simulink model "Versuch_1 (1)"  (R2022b)
settings: Solver=VariableStepAuto  StartTime=0.0  StopTime=inf  MaxStep=0.00001  RelTol=1e-3
libraries: simulink_extras x2, simulink x2
settings Model: Creator=mouaz  LastModifiedBy=mouaz

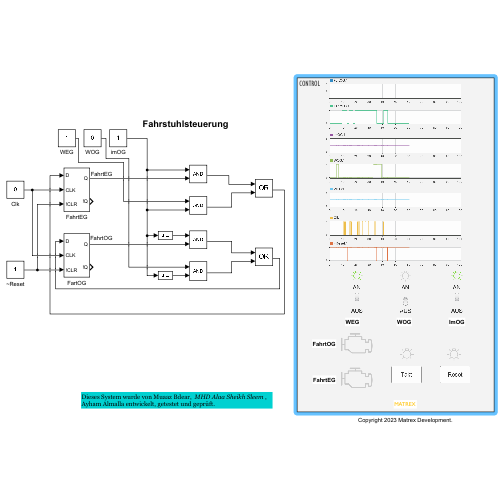
[thumbnail: Simulink's stored preview of the top-level diagram]
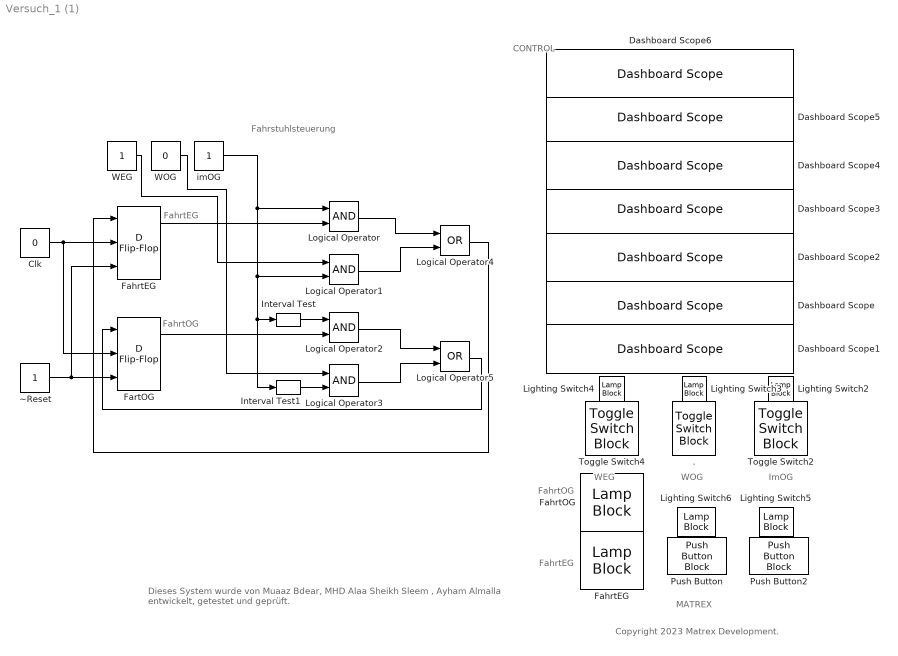
== system Versuch_1 (1) ==
  note: MATREX
  note: FahrtOG
  note: WEG
  note: FahrtEG
  note: FahrtOG
  note: WOG
  note: ImOG
  note: FahrtEG
  note: CONTROL
  note: Fahrstuhlsteuerung
  note: Copyright 2023 Matrex Development.
  note: Dieses System wurde von Muaaz Bdear, MHD Alaa Sheikh Sleem , Ayham Almalla entwickelt, getestet und geprüft.
  " FahrtEG" : LampBlock  LabelPosition=Hide  Icon=Engine
  . : ToggleSwitchBlock  LabelPosition=Hide
      settings: Values={{'AUS', 'AN'}, [0 1]}
  Clk : Constant  Value=0
  Dashboard Scope{,1..6} (7 alike) : DashboardScope
  FahrtEG : simulink_extras/Flip Flops/D Flip-Flop
  FahrtOG : LampBlock  LabelPosition=Hide  Icon=Engine
  FartOG : simulink_extras/Flip Flops/D Flip-Flop
  Interval Test : simulink/Logic and Bit Operations/Interval Test  IntervalClosedRight=on  uplimit=0.5  IntervalClosedLeft=on  lowlimit=-0.5  OutDataTypeStr=boolean
  Interval Test1 : simulink/Logic and Bit Operations/Interval Test  IntervalClosedRight=on  uplimit=0.5  IntervalClosedLeft=on  lowlimit=-0.5  OutDataTypeStr=boolean
  Lighting Switch{2..6} (5 alike) : LampBlock  LabelPosition=Hide  Icon=LightingSwitch
  Logical Operator{,1..3} (4 alike) : Logic  AllPortsSameDT=off  OutDataTypeStr=boolean
  Logical Operator4 : Logic  Operator=OR  AllPortsSameDT=off  OutDataTypeStr=boolean
  Logical Operator5 : Logic  Operator=OR  AllPortsSameDT=off  OutDataTypeStr=boolean
  Push Button : PushButtonBlock  ButtonText=Takt  OffValue=0.000000
  Push Button2 : PushButtonBlock  ButtonText=Reset  OnValue=0  IconAlignment=Center  IconColor=On  OffValue=1.000000
  Toggle Switch2 : ToggleSwitchBlock  LabelPosition=Hide
      settings: Values={{'AUS', 'AN'}, [0 1]}
  Toggle Switch4 : ToggleSwitchBlock  LabelPosition=Hide
      settings: Values={{'AUS', 'AN'}, [0 1]}
  WEG : Constant
  WOG : Constant  Value=0
  imOG : Constant
  ~Reset : Constant
  wires:
  Clk/1 -> FahrtEG/2, FartOG/2
  ~Reset/1 -> FahrtEG/3, FartOG/3
  Logical Operator/1 -> Logical Operator4/1
  Logical Operator1/1 -> Logical Operator4/2
  Logical Operator2/1 -> Logical Operator5/1
  Logical Operator3/1 -> Logical Operator5/2
  Logical Operator5/1 -> FartOG/1
  Logical Operator4/1 -> FahrtEG/1
  Interval Test/1 -> Logical Operator2/1
  Interval Test1/1 -> Logical Operator3/2
  imOG/1 -> Logical Operator/1, Logical Operator1/2, Interval Test/1, Interval Test1/1
  FahrtEG/1 -> Logical Operator/2
  FartOG/1 -> Logical Operator2/2
  WOG/1 -> Logical Operator3/1
  WEG/1 -> Logical Operator1/1
